simulink model "ES259A_BattVltgCorrln"  (R2013b)
settings: Solver=FixedStepDiscrete  SolverMode=SingleTasking  StartTime=0.0  StopTime=Inf  FixedStep=0.002  RelTol=1e-3
values from neighbouring files (symbols this model uses):
  BattVltgCorrlnAllwdVltgDif = DataDict.Calibration    [ES259A_BattVltgCorrln_DataDict.m]
  BattVltgCorrlnBattLoVltg = DataDict.Calibration    [ES259A_BattVltgCorrln_DataDict.m]
  BattVltgCorrlnBattOverVltg = DataDict.Calibration    [ES259A_BattVltgCorrln_DataDict.m]
  BattVltgCorrlnBattUnderVltg = DataDict.Calibration    [ES259A_BattVltgCorrln_DataDict.m]
  BattVltgCorrlnNtc0x03C0x0440x04CFailStep = DataDict.Calibration    [ES259A_BattVltgCorrln_DataDict.m]
  BattVltgCorrlnNtc0x03C0x0440x04CPassStep = DataDict.Calibration    [ES259A_BattVltgCorrln_DataDict.m]
  BattVltgCorrlnNtc0x03DFailStep = DataDict.Calibration    [ES259A_BattVltgCorrln_DataDict.m]
  BattVltgCorrlnNtc0x03DPassStep = DataDict.Calibration    [ES259A_BattVltgCorrln_DataDict.m]
  BattVltgCorrlnNtc0x0B0FailStep = DataDict.Calibration    [ES259A_BattVltgCorrln_DataDict.m]
  BattVltgCorrlnNtc0x0B0PassStep = DataDict.Calibration    [ES259A_BattVltgCorrln_DataDict.m]
  BattVltgCorrlnNtc0x0B1FailStep = DataDict.Calibration    [ES259A_BattVltgCorrln_DataDict.m]
  BattVltgCorrlnNtc0x0B1PassStep = DataDict.Calibration    [ES259A_BattVltgCorrln_DataDict.m]
  BattVltgCorrlnNtc0x0B5FailStep = DataDict.Calibration    [ES259A_BattVltgCorrln_DataDict.m]
  BattVltgCorrlnNtc0x0B5PassStep = DataDict.Calibration    [ES259A_BattVltgCorrln_DataDict.m]
  BattVltgCorrlnRcvrlBattLoVltg = DataDict.Calibration    [ES259A_BattVltgCorrln_DataDict.m]
  BattVltgCorrlnRcvrlBattOverVltg = DataDict.Calibration    [ES259A_BattVltgCorrln_DataDict.m]
  BattVltgCorrlnRcvrlBattUnderVltg = DataDict.Calibration    [ES259A_BattVltgCorrln_DataDict.m]
  BattVltgCorrlnSysMinVltg = DataDict.ImprtdCal    [ES250A_BattVltg_DataDict.m]    (also in ES259A_BattVltgCorrln_DataDict.m = DataDict.Calibration)
  BattVltgSwdMax = DataDict.Calibration    [ES250A_BattVltg_DataDict.m]
  ELECGLBPRM_STRTUPSTPWRDISCNCTBTESTCMPL_CNT_U08 = DataDict.Constant    [ES999A_ElecGlbPrm_DataDict.m]
  SYSVLTGFLTDUALIVTR_CNT_U08 = DataDict.Constant    [ES259A_BattVltgCorrln_DataDict.m]
undefined symbols (not defined in the file or in its folder): NtcNr1, NtcSts1, SigQlfr1
libraries: simulink x14
(part 2 of 7)

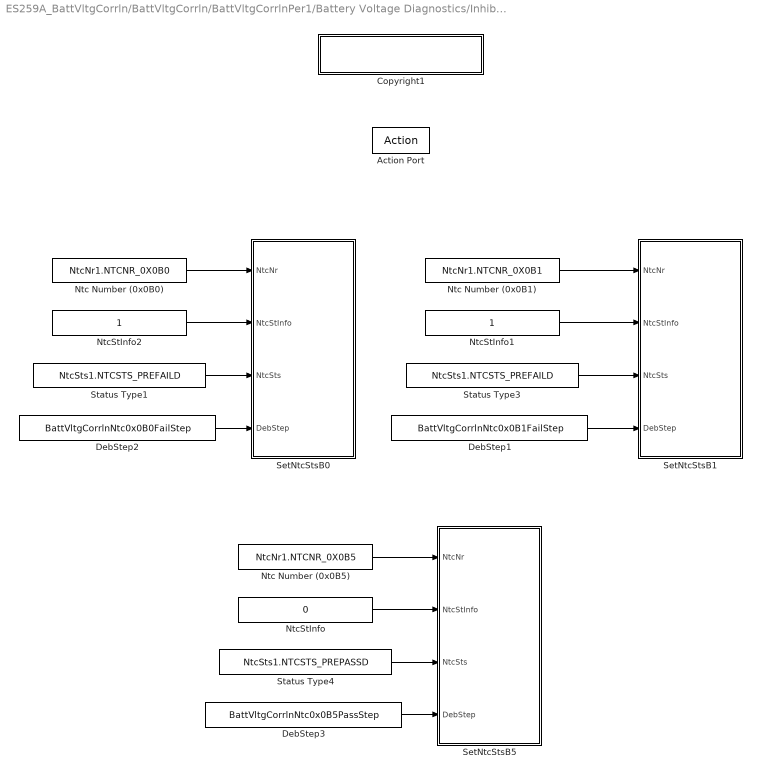
== system ES259A_BattVltgCorrln/BattVltgCorrln/BattVltgCorrlnPer1/Battery Voltage Diagnostics/Inhibition Off/BattVltg < UnderVltg ==
  Action Port : ActionPort  ActionType=elseif
  Copyright1 : Subsystem  Description=|  mask(Copyright Information){none=on}
      | Copyright info block.                                               
      |                                                                     
      | Place copyright information at the top of every subsystem in design.
      mask prompts: none "No parameters"
      mask help: Place copyright information at the top of every subsystem in design.
      mask Display:
      | NxtrConf = 'Nexteer Confidential';
      | 
      | sys = bdroot; %handle for the current model ("system")
      | first = get_param(sys,'Created');
      | if(isempty(first))
      |     first = datestr(now,'yyyy');
      | else
      |     first = first(end-3:end);  %year is last four digits
      | end
      | 
      | last = get_param(sys,'LastModifiedDate');
      | if isempty(last)
      |     last = datestr(now,'yyyy');
      | else
      |     last = last(end-3:end);
      | end
      | 
      | if strcmp(first,last)
      |     fprintf('%s\nCopyright  %s Nexteer',NxtrConf,first);
      | else
      |     fprintf('%s\n%s%s-%s Nexteer',NxtrConf,char(169),first,last);
      | end
  DebStep1 : Constant  RequirementInfo={} %GIDa_0598bf5a_aaf0_4b97_afa0_4ce885a32bb8  Value=BattVltgCorrlnNtc0x0B1FailStep
  DebStep2 : Constant  RequirementInfo={} %GIDa_685c459f_8ecf_4a50_ac99_b8f45226fa6c  Value=BattVltgCorrlnNtc0x0B0FailStep
  DebStep3 : Constant  RequirementInfo={} %GIDa_9b705539_3388_49d4_a9c4_1f9b80dca541  Value=BattVltgCorrlnNtc0x0B5PassStep
  Ntc Number (0x0B0) : Constant  RequirementInfo={} %GIDa_cf4028b3_d959_4486_ab31_c034a5ca4cc4  Value=NtcNr1.NTCNR_0X0B0
  Ntc Number (0x0B1) : Constant  RequirementInfo={} %GIDa_5f79512e_93d0_4897_819c_218087ef9b75  Value=NtcNr1.NTCNR_0X0B1
  Ntc Number (0x0B5) : Constant  RequirementInfo={} %GIDa_904ad95e_12a3_4e75_a9d8_4cbcdd417791  Value=NtcNr1.NTCNR_0X0B5
  NtcStInfo : Constant  RequirementInfo={} %GIDa_4441bbda_b41e_42a7_b756_58e3cd087cb3  Value=0
  NtcStInfo1 : Constant  RequirementInfo={} %GIDa_57252366_045e_4296_9390_0282e5b32e76
  NtcStInfo2 : Constant  RequirementInfo={} %GIDa_223941f7_8959_4cc2_be6b_aca07eb20863
  SetNtcStsB0 : Subsystem  RequirementInfo={} %GIDa_a05f2340_80be_498b_a515_3a125eea5a1c
      settings: RTWSystemCode=Inline
  SetNtcStsB1 : Subsystem  RequirementInfo={} %GIDa_2799902e_9be6_4464_9ef4_85cff93dc547
      settings: RTWSystemCode=Inline
  SetNtcStsB5 : Subsystem  RequirementInfo={} %GIDa_f69f2d5e_6d2d_47bd_a0ed_6b843557cb48
      settings: RTWSystemCode=Inline
  Status Type1 : Constant  Value=NtcSts1.NTCSTS_PREFAILD
  Status Type3 : Constant  Value=NtcSts1.NTCSTS_PREFAILD
  Status Type4 : Constant  Value=NtcSts1.NTCSTS_PREPASSD
  wires:
  DebStep3/1 -> SetNtcStsB5/4(DebStep)
  Ntc Number (0x0B5)/1 -> SetNtcStsB5/1(NtcNr)
  Status Type4/1 -> SetNtcStsB5/3(NtcSts)
  NtcStInfo/1 -> SetNtcStsB5/2(NtcStInfo)
  DebStep1/1 -> SetNtcStsB1/4(DebStep)
  Ntc Number (0x0B1)/1 -> SetNtcStsB1/1(NtcNr)
  Status Type3/1 -> SetNtcStsB1/3(NtcSts)
  NtcStInfo1/1 -> SetNtcStsB1/2(NtcStInfo)
  DebStep2/1 -> SetNtcStsB0/4(DebStep)
  Ntc Number (0x0B0)/1 -> SetNtcStsB0/1(NtcNr)
  Status Type1/1 -> SetNtcStsB0/3(NtcSts)
  NtcStInfo2/1 -> SetNtcStsB0/2(NtcStInfo)

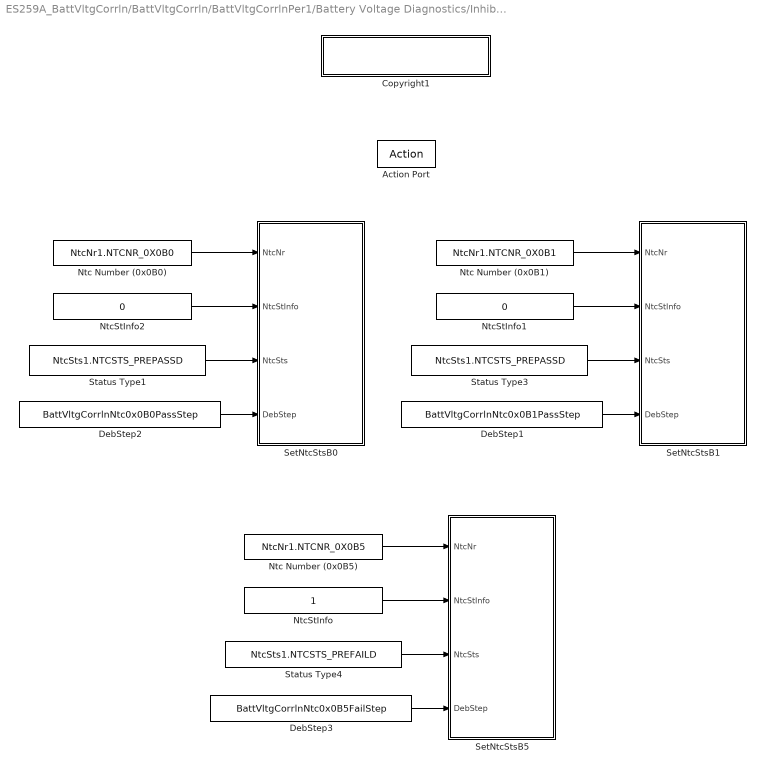
== system ES259A_BattVltgCorrln/BattVltgCorrln/BattVltgCorrlnPer1/Battery Voltage Diagnostics/Inhibition Off/BattVltg > OverVltg ==
  Action Port : ActionPort  ActionType=then
  Copyright1 : Subsystem  Description=|  mask(Copyright Information){none=on}
      | Copyright info block.                                               
      |                                                                     
      | Place copyright information at the top of every subsystem in design.
      mask prompts: none "No parameters"
      mask help: Place copyright information at the top of every subsystem in design.
      mask Display:
      | NxtrConf = 'Nexteer Confidential';
      | 
      | sys = bdroot; %handle for the current model ("system")
      | first = get_param(sys,'Created');
      | if(isempty(first))
      |     first = datestr(now,'yyyy');
      | else
      |     first = first(end-3:end);  %year is last four digits
      | end
      | 
      | last = get_param(sys,'LastModifiedDate');
      | if isempty(last)
      |     last = datestr(now,'yyyy');
      | else
      |     last = last(end-3:end);
      | end
      | 
      | if strcmp(first,last)
      |     fprintf('%s\nCopyright  %s Nexteer',NxtrConf,first);
      | else
      |     fprintf('%s\n%s%s-%s Nexteer',NxtrConf,char(169),first,last);
      | end
  DebStep1 : Constant  RequirementInfo={} %GIDa_5b68fa7b_f1e7_4ed6_9f2a_ab24fca75616  Value=BattVltgCorrlnNtc0x0B1PassStep
  DebStep2 : Constant  RequirementInfo={} %GIDa_191f3c4e_21e3_474b_b55c_a731c76d754d  Value=BattVltgCorrlnNtc0x0B0PassStep
  DebStep3 : Constant  RequirementInfo={} %GIDa_2c88b3f9_04c3_4280_9b15_076fd79c73eb  Value=BattVltgCorrlnNtc0x0B5FailStep
  Ntc Number (0x0B0) : Constant  RequirementInfo={} %GIDa_bb719727_cb42_4cb9_b9e3_a08eebbae508  Value=NtcNr1.NTCNR_0X0B0
  Ntc Number (0x0B1) : Constant  RequirementInfo={} %GIDa_6c95452a_896b_4c54_a654_f48e1e2d355a  Value=NtcNr1.NTCNR_0X0B1
  Ntc Number (0x0B5) : Constant  RequirementInfo={} %GIDa_721d6e88_627b_4e2f_8f46_913da58a843e  Value=NtcNr1.NTCNR_0X0B5
  NtcStInfo : Constant  RequirementInfo={} %GIDa_827cc2be_693a_43f1_b3e2_73fbee37a14d
  NtcStInfo1 : Constant  RequirementInfo={} %GIDa_bca492a7_1662_4888_ad8d_ae6b1dae183a  Value=0
  NtcStInfo2 : Constant  RequirementInfo={} %GIDa_7b0402a1_1968_4edc_a9d0_b1daf546780e  Value=0
  SetNtcStsB0 : Subsystem  RequirementInfo={} %GIDa_1b24742d_05be_4c4b_8fc0_dd66dcf1280b
      settings: RTWSystemCode=Inline
  SetNtcStsB1 : Subsystem  RequirementInfo={} %GIDa_c679b03b_02ce_426b_9f30_dcd3afd0a8aa
      settings: RTWSystemCode=Inline
  SetNtcStsB5 : Subsystem  RequirementInfo={} %GIDa_31e42cdd_bb57_47a8_812e_9b9b6d257680
      settings: RTWSystemCode=Inline
  Status Type1 : Constant  Value=NtcSts1.NTCSTS_PREPASSD
  Status Type3 : Constant  Value=NtcSts1.NTCSTS_PREPASSD
  Status Type4 : Constant  Value=NtcSts1.NTCSTS_PREFAILD
  wires:
  DebStep3/1 -> SetNtcStsB5/4(DebStep)
  Ntc Number (0x0B5)/1 -> SetNtcStsB5/1(NtcNr)
  Status Type4/1 -> SetNtcStsB5/3(NtcSts)
  NtcStInfo/1 -> SetNtcStsB5/2(NtcStInfo)
  DebStep1/1 -> SetNtcStsB1/4(DebStep)
  Ntc Number (0x0B1)/1 -> SetNtcStsB1/1(NtcNr)
  Status Type3/1 -> SetNtcStsB1/3(NtcSts)
  NtcStInfo1/1 -> SetNtcStsB1/2(NtcStInfo)
  DebStep2/1 -> SetNtcStsB0/4(DebStep)
  Ntc Number (0x0B0)/1 -> SetNtcStsB0/1(NtcNr)
  Status Type1/1 -> SetNtcStsB0/3(NtcSts)
  NtcStInfo2/1 -> SetNtcStsB0/2(NtcStInfo)

== system ES259A_BattVltgCorrln/BattVltgCorrln/BattVltgCorrlnPer1/Battery Voltage Diagnostics/Inhibition Off/Copyright1 ==

== system ES259A_BattVltgCorrln/BattVltgCorrln/BattVltgCorrlnPer1/Battery Voltage Diagnostics/Inhibition Off/LowVltg <= Batt <= OverVltg ==
  BattVltg : Inport
  Action Port : ActionPort  ActionType=else
  Constant3 : Constant  Value=BattVltgCorrlnRcvrlBattLoVltg
  Constant4 : Constant  Value=BattVltgCorrlnRcvrlBattOverVltg
  Copyright1 : Subsystem  Description=|  mask(Copyright Information){none=on}
      | Copyright info block.                                               
      |                                                                     
      | Place copyright information at the top of every subsystem in design.
      mask prompts: none "No parameters"
      mask help: Place copyright information at the top of every subsystem in design.
      mask Display:
      | NxtrConf = 'Nexteer Confidential';
      | 
      | sys = bdroot; %handle for the current model ("system")
      | first = get_param(sys,'Created');
      | if(isempty(first))
      |     first = datestr(now,'yyyy');
      | else
      |     first = first(end-3:end);  %year is last four digits
      | end
      | 
      | last = get_param(sys,'LastModifiedDate');
      | if isempty(last)
      |     last = datestr(now,'yyyy');
      | else
      |     last = last(end-3:end);
      | end
      | 
      | if strcmp(first,last)
      |     fprintf('%s\nCopyright  %s Nexteer',NxtrConf,first);
      | else
      |     fprintf('%s\n%s%s-%s Nexteer',NxtrConf,char(169),first,last);
      | end
  If : If  NumInputs=3  IfExpression=u1 < u2  ElseIfExpressions=u1 > u3
  If Action : Subsystem  RequirementInfo={} %GIDa_b1af21bc_9eb4_417c_a100_6df68644121f
  If Action 1 : Subsystem  RequirementInfo={} %GIDa_2aefb21e_eb07_4191_90dd_ce534c812ab2
  No Fault Condition : Subsystem  RequirementInfo={} %GIDa_69801dee_7fa5_43b7_a6cc_99eb8f83c948
  wires:
  BattVltg/1 -> If/1
  If/2 -> If Action 1/Action
  If/1 -> If Action/Action
  Constant3/1 -> If/2
  If/3 -> No Fault Condition/Action
  Constant4/1 -> If/3

== system ES259A_BattVltgCorrln/BattVltgCorrln/BattVltgCorrlnPer1/Battery Voltage Diagnostics/Inhibition Off/UnderVltg <= BattVltg < LowVltg ==
  BattVltg : Inport
  Action Port : ActionPort  ActionType=elseif
  Constant5 : Constant  Value=BattVltgCorrlnRcvrlBattUnderVltg
  Copyright1 : Subsystem  Description=|  mask(Copyright Information){none=on}
      | Copyright info block.                                               
      |                                                                     
      | Place copyright information at the top of every subsystem in design.
      mask prompts: none "No parameters"
      mask help: Place copyright information at the top of every subsystem in design.
      mask Display:
      | NxtrConf = 'Nexteer Confidential';
      | 
      | sys = bdroot; %handle for the current model ("system")
      | first = get_param(sys,'Created');
      | if(isempty(first))
      |     first = datestr(now,'yyyy');
      | else
      |     first = first(end-3:end);  %year is last four digits
      | end
      | 
      | last = get_param(sys,'LastModifiedDate');
      | if isempty(last)
      |     last = datestr(now,'yyyy');
      | else
      |     last = last(end-3:end);
      | end
      | 
      | if strcmp(first,last)
      |     fprintf('%s\nCopyright  %s Nexteer',NxtrConf,first);
      | else
      |     fprintf('%s\n%s%s-%s Nexteer',NxtrConf,char(169),first,last);
      | end
  If : If  NumInputs=2  IfExpression=u1 < u2
  If Action : Subsystem  RequirementInfo={} %GIDa_369088cf_da79_4a28_9862_390f58b5a948
  If Action 1 : Subsystem  RequirementInfo={} %GIDa_0ff1494d_f51e_44a9_8e1c_01ce1d304446
  wires:
  BattVltg/1 -> If/1
  Constant5/1 -> If/2
  If/2 -> If Action 1/Action
  If/1 -> If Action/Action

== system ES259A_BattVltgCorrln/BattVltgCorrln/BattVltgCorrlnPer1/Battery Voltage Diagnostics/Inhibition On/Copyright1 ==

== system ES259A_BattVltgCorrln/BattVltgCorrln/BattVltgCorrlnPer1/WarmInit or Enable/Determine Correlation Status/Copyright1 ==

== system ES259A_BattVltgCorrln/BattVltgCorrln/BattVltgCorrlnPer1/WarmInit or Enable/Determine Correlation Status/Use Arbitraiton Voltage ==
  Action Port : ActionPort  ActionType=else
  Constant : Constant  Value=0  OutDataTypeStr=boolean
  Copyright1 : Subsystem  Description=|  mask(Copyright Information){none=on}
      | Copyright info block.                                               
      |                                                                     
      | Place copyright information at the top of every subsystem in design.
      mask prompts: none "No parameters"
      mask help: Place copyright information at the top of every subsystem in design.
      mask Display:
      | NxtrConf = 'Nexteer Confidential';
      | 
      | sys = bdroot; %handle for the current model ("system")
      | first = get_param(sys,'Created');
      | if(isempty(first))
      |     first = datestr(now,'yyyy');
      | else
      |     first = first(end-3:end);  %year is last four digits
      | end
      | 
      | last = get_param(sys,'LastModifiedDate');
      | if isempty(last)
      |     last = datestr(now,'yyyy');
      | else
      |     last = last(end-3:end);
      | end
      | 
      | if strcmp(first,last)
      |     fprintf('%s\nCopyright  %s Nexteer',NxtrConf,first);
      | else
      |     fprintf('%s\n%s%s-%s Nexteer',NxtrConf,char(169),first,last);
      | end
  DftBrdgVltgActv : Outport
  wires:
  Constant/1 -> DftBrdgVltgActv/1

== system ES259A_BattVltgCorrln/BattVltgCorrln/BattVltgCorrlnPer1/WarmInit or Enable/Determine Correlation Status/Use Default Voltage ==
  Action Port : ActionPort  ActionType=then
  Constant : Constant  OutDataTypeStr=boolean
  Copyright1 : Subsystem  Description=|  mask(Copyright Information){none=on}
      | Copyright info block.                                               
      |                                                                     
      | Place copyright information at the top of every subsystem in design.
      mask prompts: none "No parameters"
      mask help: Place copyright information at the top of every subsystem in design.
      mask Display:
      | NxtrConf = 'Nexteer Confidential';
      | 
      | sys = bdroot; %handle for the current model ("system")
      | first = get_param(sys,'Created');
      | if(isempty(first))
      |     first = datestr(now,'yyyy');
      | else
      |     first = first(end-3:end);  %year is last four digits
      | end
      | 
      | last = get_param(sys,'LastModifiedDate');
      | if isempty(last)
      |     last = datestr(now,'yyyy');
      | else
      |     last = last(end-3:end);
      | end
      | 
      | if strcmp(first,last)
      |     fprintf('%s\nCopyright  %s Nexteer',NxtrConf,first);
      | else
      |     fprintf('%s\n%s%s-%s Nexteer',NxtrConf,char(169),first,last);
      | end
  DftBrdgVltgActv : Outport
  wires:
  Constant/1 -> DftBrdgVltgActv/1

== system ES259A_BattVltgCorrln/BattVltgCorrln/BattVltgCorrlnPer1/WarmInit or Enable/Determine Independent Signals/BattVltg Failed ==
  Action Port : ActionPort  ActionType=else
  Copyright1 : Subsystem  Description=|  mask(Copyright Information){none=on}
      | Copyright info block.                                               
      |                                                                     
      | Place copyright information at the top of every subsystem in design.
      mask prompts: none "No parameters"
      mask help: Place copyright information at the top of every subsystem in design.
      mask Display:
      | NxtrConf = 'Nexteer Confidential';
      | 
      | sys = bdroot; %handle for the current model ("system")
      | first = get_param(sys,'Created');
      | if(isempty(first))
      |     first = datestr(now,'yyyy');
      | else
      |     first = first(end-3:end);  %year is last four digits
      | end
      | 
      | last = get_param(sys,'LastModifiedDate');
      | if isempty(last)
      |     last = datestr(now,'yyyy');
      | else
      |     last = last(end-3:end);
      | end
      | 
      | if strcmp(first,last)
      |     fprintf('%s\nCopyright  %s Nexteer',NxtrConf,first);
      | else
      |     fprintf('%s\n%s%s-%s Nexteer',NxtrConf,char(169),first,last);
      | end
  Failed : Constant  Value=0  OutDataTypeStr=uint8
  BattVltgNotFailed : Outport
  wires:
  Failed/1 -> BattVltgNotFailed/1

== system ES259A_BattVltgCorrln/BattVltgCorrln/BattVltgCorrlnPer1/WarmInit or Enable/Determine Independent Signals/BattVltg Passed ==
  Action Port : ActionPort  ActionType=then
  Copyright1 : Subsystem  Description=|  mask(Copyright Information){none=on}
      | Copyright info block.                                               
      |                                                                     
      | Place copyright information at the top of every subsystem in design.
      mask prompts: none "No parameters"
      mask help: Place copyright information at the top of every subsystem in design.
      mask Display:
      | NxtrConf = 'Nexteer Confidential';
      | 
      | sys = bdroot; %handle for the current model ("system")
      | first = get_param(sys,'Created');
      | if(isempty(first))
      |     first = datestr(now,'yyyy');
      | else
      |     first = first(end-3:end);  %year is last four digits
      | end
      | 
      | last = get_param(sys,'LastModifiedDate');
      | if isempty(last)
      |     last = datestr(now,'yyyy');
      | else
      |     last = last(end-3:end);
      | end
      | 
      | if strcmp(first,last)
      |     fprintf('%s\nCopyright  %s Nexteer',NxtrConf,first);
      | else
      |     fprintf('%s\n%s%s-%s Nexteer',NxtrConf,char(169),first,last);
      | end
  Passed : Constant  OutDataTypeStr=uint8
  BattVltgNotFailed : Outport
  wires:
  Passed/1 -> BattVltgNotFailed/1

== system ES259A_BattVltgCorrln/BattVltgCorrln/BattVltgCorrlnPer1/WarmInit or Enable/Determine Independent Signals/BattVltgSwd1 Failed ==
  Action Port : ActionPort  ActionType=else
  Copyright1 : Subsystem  Description=|  mask(Copyright Information){none=on}
      | Copyright info block.                                               
      |                                                                     
      | Place copyright information at the top of every subsystem in design.
      mask prompts: none "No parameters"
      mask help: Place copyright information at the top of every subsystem in design.
      mask Display:
      | NxtrConf = 'Nexteer Confidential';
      | 
      | sys = bdroot; %handle for the current model ("system")
      | first = get_param(sys,'Created');
      | if(isempty(first))
      |     first = datestr(now,'yyyy');
      | else
      |     first = first(end-3:end);  %year is last four digits
      | end
      | 
      | last = get_param(sys,'LastModifiedDate');
      | if isempty(last)
      |     last = datestr(now,'yyyy');
      | else
      |     last = last(end-3:end);
      | end
      | 
      | if strcmp(first,last)
      |     fprintf('%s\nCopyright  %s Nexteer',NxtrConf,first);
      | else
      |     fprintf('%s\n%s%s-%s Nexteer',NxtrConf,char(169),first,last);
      | end
  Failed : Constant  Value=0  OutDataTypeStr=uint8
  BattVltgSwd1NotFailed : Outport
  wires:
  Failed/1 -> BattVltgSwd1NotFailed/1

== system ES259A_BattVltgCorrln/BattVltgCorrln/BattVltgCorrlnPer1/WarmInit or Enable/Determine Independent Signals/BattVltgSwd1 Passed ==
  Action Port : ActionPort  ActionType=then
  Copyright1 : Subsystem  Description=|  mask(Copyright Information){none=on}
      | Copyright info block.                                               
      |                                                                     
      | Place copyright information at the top of every subsystem in design.
      mask prompts: none "No parameters"
      mask help: Place copyright information at the top of every subsystem in design.
      mask Display:
      | NxtrConf = 'Nexteer Confidential';
      | 
      | sys = bdroot; %handle for the current model ("system")
      | first = get_param(sys,'Created');
      | if(isempty(first))
      |     first = datestr(now,'yyyy');
      | else
      |     first = first(end-3:end);  %year is last four digits
      | end
      | 
      | last = get_param(sys,'LastModifiedDate');
      | if isempty(last)
      |     last = datestr(now,'yyyy');
      | else
      |     last = last(end-3:end);
      | end
      | 
      | if strcmp(first,last)
      |     fprintf('%s\nCopyright  %s Nexteer',NxtrConf,first);
      | else
      |     fprintf('%s\n%s%s-%s Nexteer',NxtrConf,char(169),first,last);
      | end
  Passed : Constant  OutDataTypeStr=uint8
  BattVltgSwd1NotFailed : Outport
  wires:
  Passed/1 -> BattVltgSwd1NotFailed/1

== system ES259A_BattVltgCorrln/BattVltgCorrln/BattVltgCorrlnPer1/WarmInit or Enable/Determine Independent Signals/BattVltgSwd2 Failed ==
  Action Port : ActionPort  ActionType=else
  Copyright1 : Subsystem  Description=|  mask(Copyright Information){none=on}
      | Copyright info block.                                               
      |                                                                     
      | Place copyright information at the top of every subsystem in design.
      mask prompts: none "No parameters"
      mask help: Place copyright information at the top of every subsystem in design.
      mask Display:
      | NxtrConf = 'Nexteer Confidential';
      | 
      | sys = bdroot; %handle for the current model ("system")
      | first = get_param(sys,'Created');
      | if(isempty(first))
      |     first = datestr(now,'yyyy');
      | else
      |     first = first(end-3:end);  %year is last four digits
      | end
      | 
      | last = get_param(sys,'LastModifiedDate');
      | if isempty(last)
      |     last = datestr(now,'yyyy');
      | else
      |     last = last(end-3:end);
      | end
      | 
      | if strcmp(first,last)
      |     fprintf('%s\nCopyright  %s Nexteer',NxtrConf,first);
      | else
      |     fprintf('%s\n%s%s-%s Nexteer',NxtrConf,char(169),first,last);
      | end
  Failed : Constant  Value=0  OutDataTypeStr=uint8
  BattVltgSwd2NotFailed : Outport
  wires:
  Failed/1 -> BattVltgSwd2NotFailed/1

== system ES259A_BattVltgCorrln/BattVltgCorrln/BattVltgCorrlnPer1/WarmInit or Enable/Determine Independent Signals/BattVltgSwd2 Passed ==
  Action Port : ActionPort  ActionType=then
  Copyright1 : Subsystem  Description=|  mask(Copyright Information){none=on}
      | Copyright info block.                                               
      |                                                                     
      | Place copyright information at the top of every subsystem in design.
      mask prompts: none "No parameters"
      mask help: Place copyright information at the top of every subsystem in design.
      mask Display:
      | NxtrConf = 'Nexteer Confidential';
      | 
      | sys = bdroot; %handle for the current model ("system")
      | first = get_param(sys,'Created');
      | if(isempty(first))
      |     first = datestr(now,'yyyy');
      | else
      |     first = first(end-3:end);  %year is last four digits
      | end
      | 
      | last = get_param(sys,'LastModifiedDate');
      | if isempty(last)
      |     last = datestr(now,'yyyy');
      | else
      |     last = last(end-3:end);
      | end
      | 
      | if strcmp(first,last)
      |     fprintf('%s\nCopyright  %s Nexteer',NxtrConf,first);
      | else
      |     fprintf('%s\n%s%s-%s Nexteer',NxtrConf,char(169),first,last);
      | end
  Passed : Constant  OutDataTypeStr=uint8
  BattVltgSwd2NotFailed : Outport
  wires:
  Passed/1 -> BattVltgSwd2NotFailed/1

== system ES259A_BattVltgCorrln/BattVltgCorrln/BattVltgCorrlnPer1/WarmInit or Enable/Determine Independent Signals/Copyright1 ==

== system ES259A_BattVltgCorrln/BattVltgCorrln/BattVltgCorrlnPer1/WarmInit or Enable/Determine Independent Signals/Diagnose Inputs ==
  BattVltgOk : Inport
  BattVltgSwd1Ok : Inport  Port=2
  BattVltgSwd2Ok : Inport  Port=3
  DiagcStsIvtr1Inactv : Inport  Port=4
  DiagcStsIvtr2Inactv : Inport  Port=5
  Copyright1 : Subsystem  Description=|  mask(Copyright Information){none=on}
      | Copyright info block.                                               
      |                                                                     
      | Place copyright information at the top of every subsystem in design.
      mask prompts: none "No parameters"
      mask help: Place copyright information at the top of every subsystem in design.
      mask Display:
      | NxtrConf = 'Nexteer Confidential';
      | 
      | sys = bdroot; %handle for the current model ("system")
      | first = get_param(sys,'Created');
      | if(isempty(first))
      |     first = datestr(now,'yyyy');
      | else
      |     first = first(end-3:end);  %year is last four digits
      | end
      | 
      | last = get_param(sys,'LastModifiedDate');
      | if isempty(last)
      |     last = datestr(now,'yyyy');
      | else
      |     last = last(end-3:end);
      | end
      | 
      | if strcmp(first,last)
      |     fprintf('%s\nCopyright  %s Nexteer',NxtrConf,first);
      | else
      |     fprintf('%s\n%s%s-%s Nexteer',NxtrConf,char(169),first,last);
      | end
  Data Store Write : DataStoreWrite  DataStoreName=dBattVltgCorrlnNtc0x03CQlfrSts
  Data Store Write1 : DataStoreWrite  DataStoreName=dBattVltgCorrlnNtc0x044QlfrSts
  Data Store Write2 : DataStoreWrite  DataStoreName=dBattVltgCorrlnNtc0x04CQlfrSts
  NTC 3C : Subsystem
  NTC 3D : Subsystem  RequirementInfo="{'linktype_rmi_doors' '0000cf46 (/ESG Group/FDD Module Requirements/EA4 Specific/ES259A_BattVltgCorrln)' '#ES259A_205' 'true' 'REQ:  ES259A_205' '' ; 'linktype_rmi_doors' '0000cf46 (/ESG Group/FDD Module Requirements/EA4 Specific/ES259A_BattVltgCorrln)' '#ES259A_207' 'true' 'REQ:  ES259A_207' '' ; 'linktype_rmi_doors' '0000cf46 (/ESG Group/FDD Module Requirements/EA4 Specific/ES259A_BattVltgCorrln)' '#ES259A_208' 'true' 'REQ:  ES259A_208' '' ; 'linktype_rmi_doors' '0000cf46 (/ESG Group/FDD Module Requirements/EA4 Specific/ES259A_BattVltgCorrln)' '#ES259A_118' 'true' 'REQ:  ES259A_118' '' ; 'linktype_rmi_doors' '0000cf46 (/ESG Group/FDD Module Requirements/EA4 Specific/ES259A_BattVltgCorrln)' '#ES259A_211' 'true' 'REQ:  ES259A_211' '' } %GIDa_dff272c8_10d1_4674_a0f7_3a56d7eab18a"
  NTC 44 : Subsystem  RequirementInfo={} %GIDa_d7a9d0c8_56a2_40b5_bce6_f08b5f761d33
  NTC 4C : Subsystem  RequirementInfo={} %GIDa_c1e3e797_604b_431e_b21e_f5385736e033
  Ntc0x03CQlfrSts : Outport
  Ntc0x044QlfrSts : Outport  Port=2
  Ntc0x04CQlfrSts : Outport  Port=3
  wires:
  NTC 44/1(Ntc0x044QlfrSts) -> Data Store Write1/1, Ntc0x044QlfrSts/1
  NTC 4C/1(Ntc0x04CQlfrSts) -> Data Store Write2/1, Ntc0x04CQlfrSts/1
  BattVltgOk/1 -> NTC 3D/1(BattVltgOk), NTC 3C/1(BattVltgOk)
  DiagcStsIvtr1Inactv/1 -> NTC 44/2(DiagcStsIvtr1Inactv)
  BattVltgSwd1Ok/1 -> NTC 3D/2(BattVltgSwd1Ok), NTC 44/1(BattVltgSwd1Ok)
  BattVltgSwd2Ok/1 -> NTC 3D/3(BattVltgSwd2Ok), NTC 4C/1(BattVltgSwd2Ok)
  DiagcStsIvtr2Inactv/1 -> NTC 4C/2(DiagcStsIvtr2Inactv)
  NTC 3C/1(Ntc0x03CQlfrSts) -> Data Store Write/1, Ntc0x03CQlfrSts/1

== system ES259A_BattVltgCorrln/BattVltgCorrln/BattVltgCorrlnPer1/WarmInit or Enable/Determine Independent Signals/Use Arbitraiton Voltage ==
  IdptSig : Inport
  Action Port : ActionPort  ActionType=else
  Copyright1 : Subsystem  Description=|  mask(Copyright Information){none=on}
      | Copyright info block.                                               
      |                                                                     
      | Place copyright information at the top of every subsystem in design.
      mask prompts: none "No parameters"
      mask help: Place copyright information at the top of every subsystem in design.
      mask Display:
      | NxtrConf = 'Nexteer Confidential';
      | 
      | sys = bdroot; %handle for the current model ("system")
      | first = get_param(sys,'Created');
      | if(isempty(first))
      |     first = datestr(now,'yyyy');
      | else
      |     first = first(end-3:end);  %year is last four digits
      | end
      | 
      | last = get_param(sys,'LastModifiedDate');
      | if isempty(last)
      |     last = datestr(now,'yyyy');
      | else
      |     last = last(end-3:end);
      | end
      | 
      | if strcmp(first,last)
      |     fprintf('%s\nCopyright  %s Nexteer',NxtrConf,first);
      | else
      |     fprintf('%s\n%s%s-%s Nexteer',NxtrConf,char(169),first,last);
      | end
  BattVltgCorrlnIdptSig : Outport
  wires:
  IdptSig/1 -> BattVltgCorrlnIdptSig/1

== system ES259A_BattVltgCorrln/BattVltgCorrln/BattVltgCorrlnPer1/WarmInit or Enable/Determine Independent Signals/Use Default Voltage ==
  Action Port : ActionPort  ActionType=then
  Constant1 : Constant  Value=0  OutDataTypeStr=uint8
  Copyright1 : Subsystem  Description=|  mask(Copyright Information){none=on}
      | Copyright info block.                                               
      |                                                                     
      | Place copyright information at the top of every subsystem in design.
      mask prompts: none "No parameters"
      mask help: Place copyright information at the top of every subsystem in design.
      mask Display:
      | NxtrConf = 'Nexteer Confidential';
      | 
      | sys = bdroot; %handle for the current model ("system")
      | first = get_param(sys,'Created');
      | if(isempty(first))
      |     first = datestr(now,'yyyy');
      | else
      |     first = first(end-3:end);  %year is last four digits
      | end
      | 
      | last = get_param(sys,'LastModifiedDate');
      | if isempty(last)
      |     last = datestr(now,'yyyy');
      | else
      |     last = last(end-3:end);
      | end
      | 
      | if strcmp(first,last)
      |     fprintf('%s\nCopyright  %s Nexteer',NxtrConf,first);
      | else
      |     fprintf('%s\n%s%s-%s Nexteer',NxtrConf,char(169),first,last);
      | end
  BattVltgCorrlnIdptSig : Outport
  wires:
  Constant1/1 -> BattVltgCorrlnIdptSig/1

== system ES259A_BattVltgCorrln/BattVltgCorrln/BattVltgCorrlnPer1/WarmInit or Enable/Instantaneous Correlation/Copyright1 ==

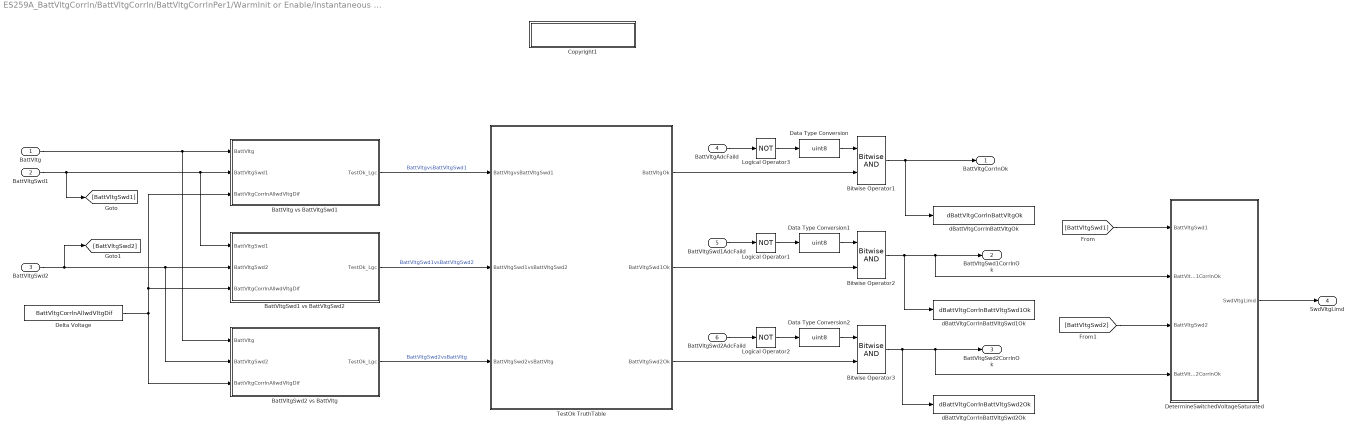
== system ES259A_BattVltgCorrln/BattVltgCorrln/BattVltgCorrlnPer1/WarmInit or Enable/Instantaneous Correlation/Correlation Check ==
  BattVltg : Inport
  BattVltgSwd1 : Inport  Port=2
  BattVltgSwd2 : Inport  Port=3
  BattVltgAdcFaild : Inport  Port=4
  BattVltgSwd1AdcFaild : Inport  Port=5
  BattVltgSwd2AdcFaild : Inport  Port=6
  BattVltg vs BattVltgSwd1 : Subsystem  RequirementInfo={} %GIDa_9616cae4_fd23_4a9e_9b47_3fcbc371c0a9  TreatAsAtomicUnit=on
  BattVltgSwd1 vs BattVltgSwd2 : Subsystem  RequirementInfo={} %GIDa_3cd37f85_ee36_4679_b9ee_187cf929014e  TreatAsAtomicUnit=on
  BattVltgSwd2 vs BattVltg : Subsystem  RequirementInfo={} %GIDa_e56f6c40_cec9_424c_9c55_9165d52d8a0f  TreatAsAtomicUnit=on
  Bitwise Operator1 : simulink/Logic and Bit Operations/Bitwise Operator  logicop=AND  UseBitMask=off  NumInputPorts=2  BitMask=bin2dec('11011001')  BitMaskRealWorld=Stored Integer
  Bitwise Operator2 : simulink/Logic and Bit Operations/Bitwise Operator  logicop=AND  UseBitMask=off  NumInputPorts=2  BitMask=bin2dec('11011001')  BitMaskRealWorld=Stored Integer
  Bitwise Operator3 : simulink/Logic and Bit Operations/Bitwise Operator  logicop=AND  UseBitMask=off  NumInputPorts=2  BitMask=bin2dec('11011001')  BitMaskRealWorld=Stored Integer
  Copyright1 : Subsystem  Description=|  mask(Copyright Information){none=on}
      | Copyright info block.                                               
      |                                                                     
      | Place copyright information at the top of every subsystem in design.
      mask prompts: none "No parameters"
      mask help: Place copyright information at the top of every subsystem in design.
      mask Display:
      | NxtrConf = 'Nexteer Confidential';
      | 
      | sys = bdroot; %handle for the current model ("system")
      | first = get_param(sys,'Created');
      | if(isempty(first))
      |     first = datestr(now,'yyyy');
      | else
      |     first = first(end-3:end);  %year is last four digits
      | end
      | 
      | last = get_param(sys,'LastModifiedDate');
      | if isempty(last)
      |     last = datestr(now,'yyyy');
      | else
      |     last = last(end-3:end);
      | end
      | 
      | if strcmp(first,last)
      |     fprintf('%s\nCopyright  %s Nexteer',NxtrConf,first);
      | else
      |     fprintf('%s\n%s%s-%s Nexteer',NxtrConf,char(169),first,last);
      | end
  Data Type Conversion : DataTypeConversion  OutDataTypeStr=uint8
  Data Type Conversion1 : DataTypeConversion  OutDataTypeStr=uint8
  Data Type Conversion2 : DataTypeConversion  OutDataTypeStr=uint8
  Delta Voltage : Constant  Value=BattVltgCorrlnAllwdVltgDif
  DetermineSwitchedVoltageSaturated : Subsystem  RequirementInfo="{'linktype_rmi_doors' '0000cf46 (/ESG Group/FDD Module Requirements/EA4 Specific/ES259A_BattVltgCorrln)' '#ES259A_152' 'true' 'REQ:  ES259A_152' '' ; 'linktype_rmi_doors' '0000cf46 (/ESG Group/FDD Module Requirements/EA4 Specific/ES259A_BattVltgCorrln)' '#ES259A_154' 'true' 'REQ:  ES259A_154' '' ; 'linktype_rmi_doors' '0000cf46 (/ESG Group/FDD Module Requirements/EA4 Specific/ES259A_BattVltgCorrln)' '#ES259A_153' 'true' 'REQ:  ES259A_153' '' ; 'linktype_rmi_doors' '0000cf46 (/ESG Group/FDD Module Requirements/EA4 Specific/ES259A_BattVltgCorrln)' '#ES259A_155' 'true' 'REQ:  ES259A_155' '' } %GIDa_6fd35311_f272_4376_b806_0dadf0e9a8a9"
  Logical Operator1 : Logic  Operator=NOT  AllPortsSameDT=off  OutDataTypeStr=boolean
  Logical Operator2 : Logic  Operator=NOT  AllPortsSameDT=off  OutDataTypeStr=boolean
  Logical Operator3 : Logic  Operator=NOT  AllPortsSameDT=off  OutDataTypeStr=boolean
  TestOk TruthTable : Truth Table  RequirementInfo={} %GIDa_c57a43f4_c002_43df_929f_b7b2d5815781  TreatAsAtomicUnit=on
  dBattVltgCorrlnBattVltgOk : DataStoreWrite  DataStoreName=dBattVltgCorrlnBattVltgOk
  dBattVltgCorrlnBattVltgSwd1Ok : DataStoreWrite  DataStoreName=dBattVltgCorrlnBattVltgSwd1Ok
  dBattVltgCorrlnBattVltgSwd2Ok : DataStoreWrite  DataStoreName=dBattVltgCorrlnBattVltgSwd2Ok
  BattVltgCorrlnOk : Outport
  BattVltgSwd1CorrlnOk : Outport  Port=2
  BattVltgSwd2CorrlnOk : Outport  Port=3
  SwdVltgLimd : Outport  RequirementInfo={} %GIDa_48b3dd50_fae8_47f4_8539_bae00a9bd97a  Port=4
  wires:
  Data Type Conversion2/1 -> Bitwise Operator3/1
  Data Type Conversion1/1 -> Bitwise Operator2/1
  Data Type Conversion/1 -> Bitwise Operator1/1
  TestOk TruthTable/3(BattVltgSwd2Ok) -> Bitwise Operator3/2
  TestOk TruthTable/2(BattVltgSwd1Ok) -> Bitwise Operator2/2
  Bitwise Operator1/1 -> dBattVltgCorrlnBattVltgOk/1, BattVltgCorrlnOk/1
  BattVltgSwd2AdcFaild/1 -> Logical Operator2/1
  BattVltgSwd1AdcFaild/1 -> Logical Operator1/1
  BattVltgAdcFaild/1 -> Logical Operator3/1
  Bitwise Operator3/1 -> DetermineSwitchedVoltageSaturated/4(BattVltgSwd2CorrlnOk), BattVltgSwd2CorrlnOk/1, dBattVltgCorrlnBattVltgSwd2Ok/1
  BattVltgSwd2/1 -> BattVltgSwd1 vs BattVltgSwd2/2(BattVltgSwd2), BattVltgSwd2 vs BattVltg/2(BattVltgSwd2), [BattVltgSwd2]
  BattVltgSwd1 vs BattVltgSwd2/1(TestOk_Lgc) -> TestOk TruthTable/2(BattVltgSwd1vsBattVltgSwd2)  "BattVltgSwd1vsBattVltgSwd2"
  BattVltg/1 -> BattVltg vs BattVltgSwd1/1(BattVltg), BattVltgSwd2 vs BattVltg/1(BattVltg)
  BattVltg vs BattVltgSwd1/1(TestOk_Lgc) -> TestOk TruthTable/1(BattVltgvsBattVltgSwd1)  "BattVltgvsBattVltgSwd1"
  Delta Voltage/1 -> BattVltgSwd2 vs BattVltg/3(BattVltgCorrlnAllwdVltgDif), BattVltgSwd1 vs BattVltgSwd2/3(BattVltgCorrlnAllwdVltgDif), BattVltg vs BattVltgSwd1/3(BattVltgCorrlnAllwdVltgDif)
  BattVltgSwd2 vs BattVltg/1(TestOk_Lgc) -> TestOk TruthTable/3(BattVltgSwd2vsBattVltg)  "BattVltgSwd2vsBattVltg"
  BattVltgSwd1/1 -> BattVltg vs BattVltgSwd1/2(BattVltgSwd1), BattVltgSwd1 vs BattVltgSwd2/1(BattVltgSwd1), [BattVltgSwd1]
  Bitwise Operator2/1 -> DetermineSwitchedVoltageSaturated/2("BattVltgSwd1CorrlnOk "), BattVltgSwd1CorrlnOk/1, dBattVltgCorrlnBattVltgSwd1Ok/1
  TestOk TruthTable/1(BattVltgOk) -> Bitwise Operator1/2
  Logical Operator3/1 -> Data Type Conversion/1
  Logical Operator1/1 -> Data Type Conversion1/1
  Logical Operator2/1 -> Data Type Conversion2/1
  [BattVltgSwd1] -> DetermineSwitchedVoltageSaturated/1(BattVltgSwd1)
  [BattVltgSwd2] -> DetermineSwitchedVoltageSaturated/3(BattVltgSwd2)
  DetermineSwitchedVoltageSaturated/1(SwdVltgLimd) -> SwdVltgLimd/1

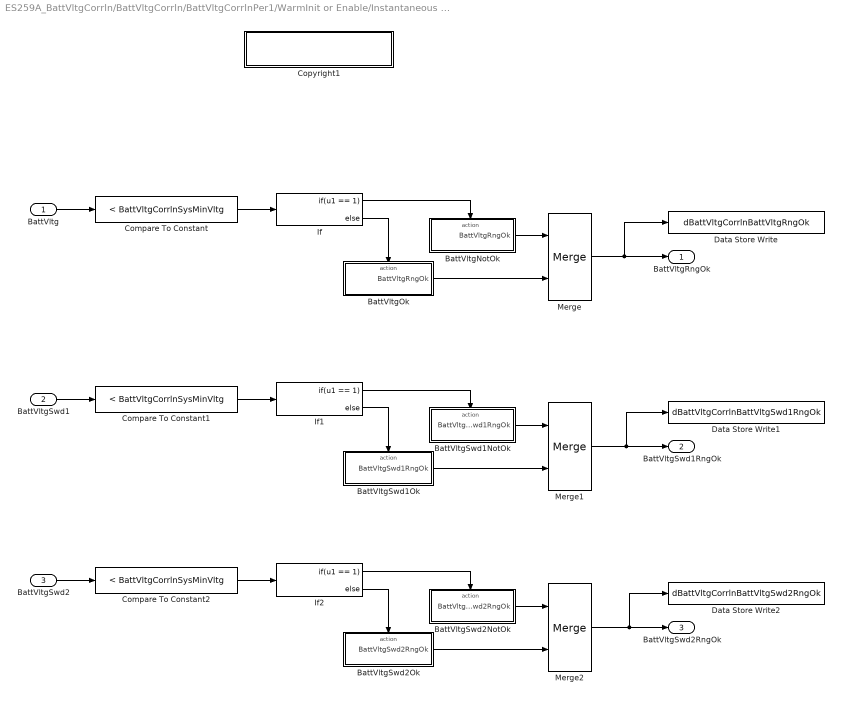
== system ES259A_BattVltgCorrln/BattVltgCorrln/BattVltgCorrlnPer1/WarmInit or Enable/Instantaneous Correlation/Range Check ==
  BattVltg : Inport
  BattVltgSwd1 : Inport  Port=2
  BattVltgSwd2 : Inport  Port=3
  BattVltgNotOk : Subsystem  TreatAsAtomicUnit=on
  BattVltgOk : Subsystem  TreatAsAtomicUnit=on
  BattVltgSwd1NotOk : Subsystem  TreatAsAtomicUnit=on
  BattVltgSwd1Ok : Subsystem  TreatAsAtomicUnit=on
  BattVltgSwd2NotOk : Subsystem  TreatAsAtomicUnit=on
  BattVltgSwd2Ok : Subsystem  TreatAsAtomicUnit=on
  Compare To Constant : simulink/Logic and Bit Operations/Compare To Constant  relop=<  const=BattVltgCorrlnSysMinVltg  OutDataTypeStr=boolean
  Compare To Constant1 : simulink/Logic and Bit Operations/Compare To Constant  relop=<  const=BattVltgCorrlnSysMinVltg  OutDataTypeStr=boolean
  Compare To Constant2 : simulink/Logic and Bit Operations/Compare To Constant  relop=<  const=BattVltgCorrlnSysMinVltg  OutDataTypeStr=boolean
  Copyright1 : Subsystem  Description=|  mask(Copyright Information){none=on}
      | Copyright info block.                                               
      |                                                                     
      | Place copyright information at the top of every subsystem in design.
      mask prompts: none "No parameters"
      mask help: Place copyright information at the top of every subsystem in design.
      mask Display:
      | NxtrConf = 'Nexteer Confidential';
      | 
      | sys = bdroot; %handle for the current model ("system")
      | first = get_param(sys,'Created');
      | if(isempty(first))
      |     first = datestr(now,'yyyy');
      | else
      |     first = first(end-3:end);  %year is last four digits
      | end
      | 
      | last = get_param(sys,'LastModifiedDate');
      | if isempty(last)
      |     last = datestr(now,'yyyy');
      | else
      |     last = last(end-3:end);
      | end
      | 
      | if strcmp(first,last)
      |     fprintf('%s\nCopyright  %s Nexteer',NxtrConf,first);
      | else
      |     fprintf('%s\n%s%s-%s Nexteer',NxtrConf,char(169),first,last);
      | end
  Data Store Write : DataStoreWrite  DataStoreName=dBattVltgCorrlnBattVltgRngOk
  Data Store Write1 : DataStoreWrite  DataStoreName=dBattVltgCorrlnBattVltgSwd1RngOk
  Data Store Write2 : DataStoreWrite  DataStoreName=dBattVltgCorrlnBattVltgSwd2RngOk
  If : If  IfExpression=u1 == 1
  If1 : If  IfExpression=u1 == 1
  If2 : If  IfExpression=u1 == 1
  Merge : Merge
  Merge1 : Merge
  Merge2 : Merge
  BattVltgRngOk : Outport
  BattVltgSwd1RngOk : Outport  Port=2
  BattVltgSwd2RngOk : Outport  Port=3
  wires:
  If2/2 -> BattVltgSwd2Ok/Action
  Merge2/1 -> Data Store Write2/1, BattVltgSwd2RngOk/1
  BattVltgSwd2NotOk/1(BattVltgSwd2RngOk) -> Merge2/1
  BattVltgSwd2Ok/1(BattVltgSwd2RngOk) -> Merge2/2
  If2/1 -> BattVltgSwd2NotOk/Action
  If1/2 -> BattVltgSwd1Ok/Action
  Merge1/1 -> Data Store Write1/1, BattVltgSwd1RngOk/1
  BattVltgSwd1NotOk/1(BattVltgSwd1RngOk) -> Merge1/1
  BattVltgSwd1Ok/1(BattVltgSwd1RngOk) -> Merge1/2
  If1/1 -> BattVltgSwd1NotOk/Action
  Merge/1 -> Data Store Write/1, BattVltgRngOk/1
  BattVltgNotOk/1(BattVltgRngOk) -> Merge/1
  BattVltgOk/1(BattVltgRngOk) -> Merge/2
  If/2 -> BattVltgOk/Action
  If/1 -> BattVltgNotOk/Action
  BattVltgSwd2/1 -> Compare To Constant2/1
  BattVltgSwd1/1 -> Compare To Constant1/1
  BattVltg/1 -> Compare To Constant/1
  Compare To Constant/1 -> If/1
  Compare To Constant1/1 -> If1/1
  Compare To Constant2/1 -> If2/1

== system ES259A_BattVltgCorrln/BattVltgCorrln/BattVltgCorrlnPer1/Battery Voltage Diagnostics/Inhibition Off/BattVltg < UnderVltg/Copyright1 ==

== system ES259A_BattVltgCorrln/BattVltgCorrln/BattVltgCorrlnPer1/Battery Voltage Diagnostics/Inhibition Off/BattVltg < UnderVltg/SetNtcStsB0 ==
  note: Only pass values 2 or 3 as input to NtcSts.
      | 2: PrePassd
      | 3: PreFaild
  NtcNr : Inport
  NtcStInfo : Inport  Port=2
  NtcSts : Inport  Port=3
  DebStep : Inport  Port=4
  Copyright1 : Subsystem  Description=|  mask(Copyright Information){none=on}
      | Copyright info block.                                               
      |                                                                     
      | Place copyright information at the top of every subsystem in design.
      mask prompts: none "No parameters"
      mask help: Place copyright information at the top of every subsystem in design.
      mask Display:
      | NxtrConf = 'Nexteer Confidential';
      | 
      | sys = bdroot; %handle for the current model ("system")
      | first = get_param(sys,'Created');
      | if(isempty(first))
      |     first = datestr(now,'yyyy');
      | else
      |     first = first(end-3:end);  %year is last four digits
      | end
      | 
      | last = get_param(sys,'LastModifiedDate');
      | if isempty(last)
      |     last = datestr(now,'yyyy');
      | else
      |     last = last(end-3:end);
      | end
      | 
      | if strcmp(first,last)
      |     fprintf('%s\nCopyright  %s Nexteer',NxtrConf,first);
      | else
      |     fprintf('%s\n%s%s-%s Nexteer',NxtrConf,char(169),first,last);
      | end
  Data Store Write1 : DataStoreWrite  RequirementInfo={} %GIDa_04a33e8c_79bb_4536_b7dc_36a8866b4c6d  DataStoreName=NtcQlfr44
  ISO Fault Debounce Design NOT TO BE IMPLEMENTED IN THIS FDD USED ONLY FOR SIMULATION PURPOSES : Stateflow chart  TreatAsAtomicUnit=on
  Only here because I could not get model to run with enumerations in the stateflow diagram : DataTypeConversion  OutDataTypeStr=uint8
  Terminator : Terminator
  Terminator1 : Terminator
  wires:
  NtcStInfo/1 -> Terminator1/1
  NtcNr/1 -> Terminator/1
  NtcSts/1 -> Only here because I could not get model to run with enumerations in the stateflow diagram/1
  DebStep/1 -> ISO Fault Debounce Design NOT TO BE IMPLEMENTED IN THIS FDD USED ONLY FOR SIMULATION PURPOSES/2(DebStep)
  Only here because I could not get model to run with enumerations in the stateflow diagram/1 -> ISO Fault Debounce Design NOT TO BE IMPLEMENTED IN THIS FDD USED ONLY FOR SIMULATION PURPOSES/1(NtcSts)
  ISO Fault Debounce Design NOT TO BE IMPLEMENTED IN THIS FDD USED ONLY FOR SIMULATION PURPOSES/1(Qualifier) -> Data Store Write1/1

== system ES259A_BattVltgCorrln/BattVltgCorrln/BattVltgCorrlnPer1/Battery Voltage Diagnostics/Inhibition Off/BattVltg < UnderVltg/SetNtcStsB1 ==
  note: Only pass values 2 or 3 as input to NtcSts.
      | 2: PrePassd
      | 3: PreFaild
  NtcNr : Inport
  NtcStInfo : Inport  Port=2
  NtcSts : Inport  Port=3
  DebStep : Inport  Port=4
  Copyright1 : Subsystem  Description=|  mask(Copyright Information){none=on}
      | Copyright info block.                                               
      |                                                                     
      | Place copyright information at the top of every subsystem in design.
      mask prompts: none "No parameters"
      mask help: Place copyright information at the top of every subsystem in design.
      mask Display:
      | NxtrConf = 'Nexteer Confidential';
      | 
      | sys = bdroot; %handle for the current model ("system")
      | first = get_param(sys,'Created');
      | if(isempty(first))
      |     first = datestr(now,'yyyy');
      | else
      |     first = first(end-3:end);  %year is last four digits
      | end
      | 
      | last = get_param(sys,'LastModifiedDate');
      | if isempty(last)
      |     last = datestr(now,'yyyy');
      | else
      |     last = last(end-3:end);
      | end
      | 
      | if strcmp(first,last)
      |     fprintf('%s\nCopyright  %s Nexteer',NxtrConf,first);
      | else
      |     fprintf('%s\n%s%s-%s Nexteer',NxtrConf,char(169),first,last);
      | end
  Data Store Write1 : DataStoreWrite  RequirementInfo={} %GIDa_6a8beded_4d4a_49f4_bcc2_b63d5b17b35f  DataStoreName=NtcQlfr44
  ISO Fault Debounce Design NOT TO BE IMPLEMENTED IN THIS FDD USED ONLY FOR SIMULATION PURPOSES : Stateflow chart  TreatAsAtomicUnit=on
  Only here because I could not get model to run with enumerations in the stateflow diagram : DataTypeConversion  OutDataTypeStr=uint8
  Terminator : Terminator
  Terminator1 : Terminator
  wires:
  NtcStInfo/1 -> Terminator1/1
  NtcNr/1 -> Terminator/1
  NtcSts/1 -> Only here because I could not get model to run with enumerations in the stateflow diagram/1
  DebStep/1 -> ISO Fault Debounce Design NOT TO BE IMPLEMENTED IN THIS FDD USED ONLY FOR SIMULATION PURPOSES/2(DebStep)
  Only here because I could not get model to run with enumerations in the stateflow diagram/1 -> ISO Fault Debounce Design NOT TO BE IMPLEMENTED IN THIS FDD USED ONLY FOR SIMULATION PURPOSES/1(NtcSts)
  ISO Fault Debounce Design NOT TO BE IMPLEMENTED IN THIS FDD USED ONLY FOR SIMULATION PURPOSES/1(Qualifier) -> Data Store Write1/1

== system ES259A_BattVltgCorrln/BattVltgCorrln/BattVltgCorrlnPer1/Battery Voltage Diagnostics/Inhibition Off/BattVltg < UnderVltg/SetNtcStsB5 ==
  note: Only pass values 2 or 3 as input to NtcSts.
      | 2: PrePassd
      | 3: PreFaild
  NtcNr : Inport
  NtcStInfo : Inport  Port=2
  NtcSts : Inport  Port=3
  DebStep : Inport  Port=4
  Copyright1 : Subsystem  Description=|  mask(Copyright Information){none=on}
      | Copyright info block.                                               
      |                                                                     
      | Place copyright information at the top of every subsystem in design.
      mask prompts: none "No parameters"
      mask help: Place copyright information at the top of every subsystem in design.
      mask Display:
      | NxtrConf = 'Nexteer Confidential';
      | 
      | sys = bdroot; %handle for the current model ("system")
      | first = get_param(sys,'Created');
      | if(isempty(first))
      |     first = datestr(now,'yyyy');
      | else
      |     first = first(end-3:end);  %year is last four digits
      | end
      | 
      | last = get_param(sys,'LastModifiedDate');
      | if isempty(last)
      |     last = datestr(now,'yyyy');
      | else
      |     last = last(end-3:end);
      | end
      | 
      | if strcmp(first,last)
      |     fprintf('%s\nCopyright  %s Nexteer',NxtrConf,first);
      | else
      |     fprintf('%s\n%s%s-%s Nexteer',NxtrConf,char(169),first,last);
      | end
  Data Store Write1 : DataStoreWrite  RequirementInfo={} %GIDa_a4eecc99_97d5_4bc1_99af_0cb6b0f0da12  DataStoreName=NtcQlfr44
  ISO Fault Debounce Design NOT TO BE IMPLEMENTED IN THIS FDD USED ONLY FOR SIMULATION PURPOSES : Stateflow chart  TreatAsAtomicUnit=on
  Only here because I could not get model to run with enumerations in the stateflow diagram : DataTypeConversion  OutDataTypeStr=uint8
  Terminator : Terminator
  Terminator1 : Terminator
  wires:
  NtcStInfo/1 -> Terminator1/1
  NtcNr/1 -> Terminator/1
  NtcSts/1 -> Only here because I could not get model to run with enumerations in the stateflow diagram/1
  DebStep/1 -> ISO Fault Debounce Design NOT TO BE IMPLEMENTED IN THIS FDD USED ONLY FOR SIMULATION PURPOSES/2(DebStep)
  Only here because I could not get model to run with enumerations in the stateflow diagram/1 -> ISO Fault Debounce Design NOT TO BE IMPLEMENTED IN THIS FDD USED ONLY FOR SIMULATION PURPOSES/1(NtcSts)
  ISO Fault Debounce Design NOT TO BE IMPLEMENTED IN THIS FDD USED ONLY FOR SIMULATION PURPOSES/1(Qualifier) -> Data Store Write1/1

== system ES259A_BattVltgCorrln/BattVltgCorrln/BattVltgCorrlnPer1/Battery Voltage Diagnostics/Inhibition Off/BattVltg > OverVltg/Copyright1 ==
